simulink subsystem "Accept_Pilot_Commands"  (R2025b)
settings: Solver=VariableStepAuto  StartTime=0.0  StopTime=10.0  RelTol=1e-3
settings Model: Creator=cdriggs  LastModifiedBy=cdriggs

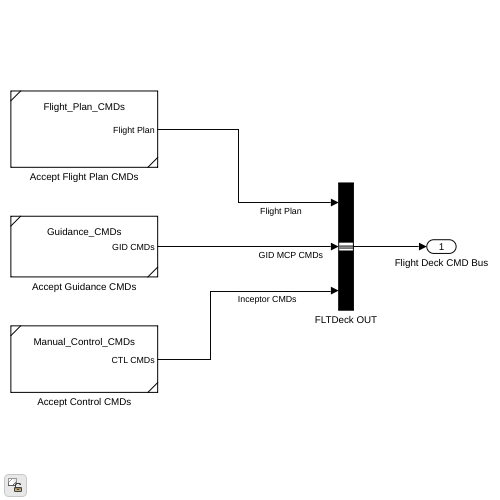
[thumbnail: Simulink's stored preview of the top-level diagram]
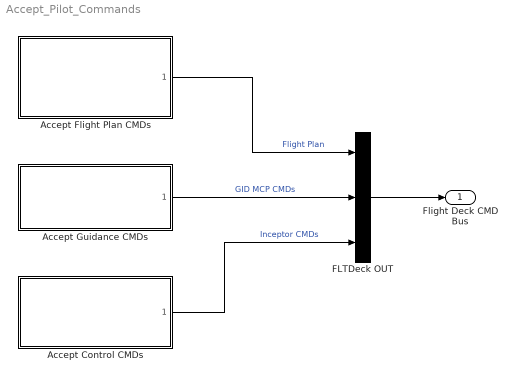
== system Accept_Pilot_Commands ==
  Accept Control CMDs : Subsystem  ReferencedSubsystem=Manual_Control_CMDs
  Accept Flight Plan CMDs : Subsystem  ReferencedSubsystem=Flight_Plan_CMDs
  Accept Guidance CMDs : Subsystem  ReferencedSubsystem=Guidance_CMDs
  FLTDeck OUT : BusCreator  Inputs=3
  Flight Deck CMD Bus : Outport
  wires:
  FLTDeck OUT/1 -> Flight Deck CMD Bus/1
  Accept Flight Plan CMDs/1 -> FLTDeck OUT/1  "Flight Plan"
  Accept Guidance CMDs/1 -> FLTDeck OUT/2  "GID MCP CMDs"
  Accept Control CMDs/1 -> FLTDeck OUT/3  "Inceptor CMDs"
